simulink model "W2Q3"  (R2020a)
settings: Solver=VariableStepAuto  StartTime=0.0  StopTime=10.0  RelTol=1e-3
values from neighbouring files (symbols this model uses):
  ki = 50    [para.m]
  kp = 1000    [para.m]
settings Model: DataDictionary=dd23.sldd  Creator=Vinayak  LastModifiedBy=Vinayak

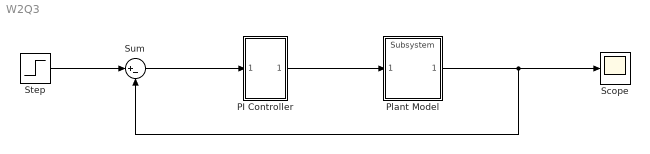
== system W2Q3 ==
  PI Controller : Subsystem
  Plant Model : ModelReference  ModelNameDialog=Subsystem  SimulationMode=Normal  ModelReferenceVersion=1.4
  Scope : Scope
  Step : Step  Time=0  After=u  SampleTime=0
  Sum : Sum  Inputs=|+-
  wires:
  PI Controller/1(Out1) -> Plant Model/1
  Plant Model/1 -> Scope/1, Sum/2
  Step/1 -> Sum/1
  Sum/1 -> PI Controller/1(In2)

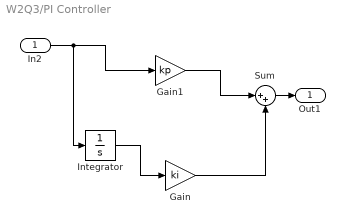
== system W2Q3/PI Controller ==
  In2 : Inport
  Gain : Gain  Gain=ki
  Gain1 : Gain  Gain=kp
  Integrator : Integrator
  Sum : Sum  Inputs=|++
  Out1 : Outport
  wires:
  In2/1 -> Integrator/1, Gain1/1
  Integrator/1 -> Gain/1
  Gain1/1 -> Sum/1
  Gain/1 -> Sum/2
  Sum/1 -> Out1/1
